simulink model "Pacemaker_Deliverable_1"  (R2025a)
settings: Solver=FixedStepAuto  StartTime=0.0  StopTime=10.0  FixedStep=1e-3  RelTol=1e-3  EnableMultiTasking=on
undefined symbols (not defined in the file): D0, D1, D10, D11, D12, D13, D2, D3, D4, D5, D6, D7, D8, D9, PTA0, PTA1, PTA2, PTB23, PTB9, PTC16, PTC17, PTC2, PTC3, PTC4, PTD0, PTD1, PTD2, PTD3
libraries: frdmk64flib x15
settings Model: ExtModeTrigDuration=5  Creator=harry  LastModifiedBy=justi
settings SolverCC: AlgebraicLoopSolver=TrustRegion
settings OptimizationCC: EnhancedBackFolding=on  PassReuseOutputArgsAs=Individual arguments  ZeroExternalMemoryAtStartup=off  ZeroInternalMemoryAtStartup=off  MaxStackSize=64  OptimizeBlockOrder=speed  DifferentSizesBufferReuse=on  OptimizationCustomize=off  EfficientTunableParamExpr=on
settings DebuggingCC: ParameterTunabilityLossMsg=error  UnconnectedInputMsg=warning  UnconnectedOutputMsg=warning  UnconnectedLineMsg=warning
settings HardwareCC: ProdBitPerPointer=32.0  ProdBitPerSizeT=32.0  ProdBitPerPtrDiffT=32.0  ProdLargestAtomicInteger=Long  ProdLargestAtomicFloat=Double  ProdWordSize=32.0  ProdHWDeviceType=ARM Compatible->ARM Cortex
settings ModelReferenceCC: EnableRefExpFcnMdlSchedulingChecks=on
settings SFSimCC: MATLABDynamicMemAlloc=off
settings RTWCC: SystemTargetFile=ert.tlc  HardwareBoard=NXP FRDM-K64F  TLCOptions="-aInlineSetEventsForThisBaseRateFcn=TLC_FALSE -aSuppressMultiTaskScheduler=TLC_FALSE  -aRateBasedStepFcn=0"  TemplateMakefile=ert_default_tmf  Toolchain=GNU Tools for ARM Embedded Processors  GPUComputeCapability=3.5  Description=Embedded Coder
settings CodeAppCC: ForceParamTrailComments=on  IgnoreCustomStorageClasses=off  OperatorAnnotations=on  SimulinkDataObjDesc=on  SFDataObjDesc=on  InsertBlockDesc=on
settings ERTTargetCC: ExtModeTransport=0.0  ExtModeStaticAlloc=off  ExtModeMexFile=ext_comm  ExtModeIntrfLevel=Level1  InlinedParameterPlacement=Hierarchical  DynamicArrayContainerType=coder::array

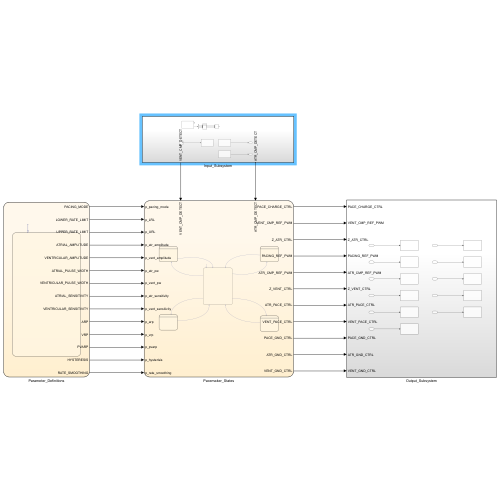
[thumbnail: Simulink's stored preview of the top-level diagram]
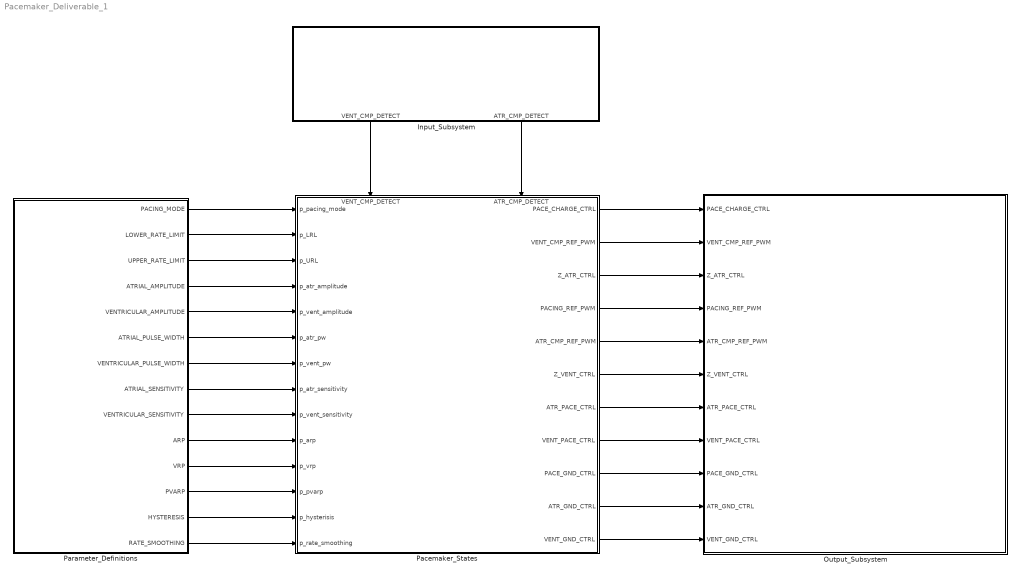
== system Pacemaker_Deliverable_1 ==
  Input_Subsystem : Subsystem
      settings: PortSchema="{\"entries\":[{\"content\":{\"sides\":[{\"content\":{\"connectorIds\":[]},\"type\":\"ConnectorPlacement.EquallySpacedRectSide\",\"uuid\":\"7aa35272-78af-4b86-b792-d4552822e5cd\"},{\"content\":{\"connectorIds\":[],\"side\":\"RIGHT\"},\"type\":\"ConnectorPlacement.EquallySpacedRectSide\",\"uuid\":\"1eeedbdd-e182-4d72-ab10-92c9b2e47973\"},{\"content\":{\"connectorIds\":[],\"side\":\"TOP\"},\"type\":\"ConnectorPlacement.EquallySpacedRectSide\",\"uuid\":\"983587ba-d25a-459a-9a3e-9f5267716506\"},{\"content\":{\"connectorIds\":[\"Out1\",\"Out2\"],\"side\":\"BOTTOM\"},\"type\":\"ConnectorPlacement.EquallySpacedRectSide\",\"uuid\":\"0cdd1530-a104-439a-8a9c-6ed3bc5e5b37\"}]},\"type\":\"ConnectorPlacement.EquallySpacedConnector\",\"uuid\":\"2c1020c0-9cac-4181-8f0f-8201f6fe3f1b\"}],\"packageUris\":[\"http://schema.mathworks.com/mf0/Connector/19700101\"],\"version\":\"1.0\"}"
  Output_Subsystem : Subsystem
  Pacemaker_States : Stateflow chart  TreatAsAtomicUnit=on
      settings: PortSchema="{\"entries\":[{\"content\":{\"sides\":[{\"content\":{\"connectorIds\":[\"In8\",\"In4\",\"In14\",\"In6\",\"In3\",\"In7\",\"In5\",\"In12\",\"In13\",\"In10\",\"In11\",\"In16\",\"In9\",\"In15\"]},\"type\":\"ConnectorPlacement.EquallySpacedRectSide\",\"uuid\":\"f7c19d4e-8469-492c-a227-d3ddaf8b11c5\"},{\"content\":{\"connectorIds\":[\"Out8\",\"Out10\",\"Out1\",\"Out7\",\"Out11\",\"Out2\",\"Out3\",\"Out4\",\"Out9\",\"Out5\",\"Out6\"],\"side\":\"RIGHT\"},\"type\":\"ConnectorPlacement.EquallySpacedRectSide\",\"uuid\":\"dec5cef5-f41f-4673-aab9-f0ca8e60eeee\"},{\"content\":{\"connectorIds\":[\"In1\",\"In2\"],\"side\":\"TOP\"},\"type\":\"ConnectorPlacement.EquallySpacedRectSide\",\"uuid\":\"d69c500f-a27d-47d0-a981-29ab2c08cb35\"}]},\"type\":\"ConnectorPlacement.EquallySpacedConnector\",\"uuid\":\"10b708de-b80e-4994-a949-6ddae67c2dfd\"}],\"packageUris\":[\"http://schema.mathworks.com/mf0/Connector/19700101\"],\"version\":\"1.0\"}"
  Parameter_Definitions : Stateflow chart  TreatAsAtomicUnit=on
      settings: PortSchema="{\"entries\":[{\"content\":{\"sides\":[{\"content\":{\"connectorIds\":[]},\"type\":\"ConnectorPlacement.EquallySpacedRectSide\",\"uuid\":\"6604c324-2550-41c6-b2f2-71f3c706ced3\"},{\"content\":{\"connectorIds\":[\"Out1\",\"Out2\",\"Out3\",\"Out4\",\"Out7\",\"Out5\",\"Out9\",\"Out8\",\"Out6\",\"Out14\",\"Out13\",\"Out12\",\"Out11\",\"Out10\"],\"side\":\"RIGHT\"},\"type\":\"ConnectorPlacement.EquallySpacedRectSide\",\"uuid\":\"7ef386a9-7013-4033-b302-df52cb7a11b5\"},{\"content\":{\"connectorIds\":[],\"side\":\"TOP\"},\"type\":\"ConnectorPlacement.EquallySpacedRectSide\",\"uuid\":\"6c75a8fc-d552-4f9b-9a9a-6aef7cb72f4d\"}]},\"type\":\"ConnectorPlacement.EquallySpacedConnector\",\"uuid\":\"c0dbf2bf-9097-47f1-93b4-de483c75bb4c\"}],\"packageUris\":[\"http://schema.mathworks.com/mf0/Connector/19700101\"],\"version\":\"1.0\"}"
  wires:
  Pacemaker_States/8(PACE_CHARGE_CTRL) -> Output_Subsystem/1(PACE_CHARGE_CTRL)
  Pacemaker_States/10(VENT_CMP_REF_PWM) -> Output_Subsystem/2(VENT_CMP_REF_PWM)
  Pacemaker_States/1(Z_ATR_CTRL) -> Output_Subsystem/3(Z_ATR_CTRL)
  Pacemaker_States/7(PACING_REF_PWM) -> Output_Subsystem/4(PACING_REF_PWM)
  Pacemaker_States/11(ATR_CMP_REF_PWM) -> Output_Subsystem/5(ATR_CMP_REF_PWM)
  Pacemaker_States/2(Z_VENT_CTRL) -> Output_Subsystem/6(Z_VENT_CTRL)
  Pacemaker_States/3(ATR_PACE_CTRL) -> Output_Subsystem/7(ATR_PACE_CTRL)
  Pacemaker_States/4(VENT_PACE_CTRL) -> Output_Subsystem/8(VENT_PACE_CTRL)
  Pacemaker_States/9(PACE_GND_CTRL) -> Output_Subsystem/9(PACE_GND_CTRL)
  Pacemaker_States/5(ATR_GND_CTRL) -> Output_Subsystem/10(ATR_GND_CTRL)
  Pacemaker_States/6(VENT_GND_CTRL) -> Output_Subsystem/11(VENT_GND_CTRL)
  Input_Subsystem/1(VENT_CMP_DETECT) -> Pacemaker_States/1(VENT_CMP_DETECT)
  Input_Subsystem/2(ATR_CMP_DETECT) -> Pacemaker_States/2(ATR_CMP_DETECT)
  Parameter_Definitions/1(PACING_MODE) -> Pacemaker_States/8(p_pacing_mode)
  Parameter_Definitions/2(LOWER_RATE_LIMIT) -> Pacemaker_States/4(p_LRL)
  Parameter_Definitions/4(ATRIAL_AMPLITUDE) -> Pacemaker_States/6(p_atr_amplitude)
  Parameter_Definitions/7(VENTRICULAR_AMPLITUDE) -> Pacemaker_States/3(p_vent_amplitude)
  Parameter_Definitions/5(ATRIAL_PULSE_WIDTH) -> Pacemaker_States/7(p_atr_pw)
  Parameter_Definitions/9(VENTRICULAR_PULSE_WIDTH) -> Pacemaker_States/5(p_vent_pw)
  Parameter_Definitions/14(ARP) -> Pacemaker_States/10(p_arp)
  Parameter_Definitions/13(VRP) -> Pacemaker_States/11(p_vrp)
  Parameter_Definitions/11(HYSTERESIS) -> Pacemaker_States/9(p_hysterisis)
  Parameter_Definitions/10(RATE_SMOOTHING) -> Pacemaker_States/15(p_rate_smoothing)
  Parameter_Definitions/8(ATRIAL_SENSITIVITY) -> Pacemaker_States/12(p_atr_sensitivity)
  Parameter_Definitions/6(VENTRICULAR_SENSITIVITY) -> Pacemaker_States/13(p_vent_sensitivity)
  Parameter_Definitions/3(UPPER_RATE_LIMIT) -> Pacemaker_States/14(p_URL)
  Parameter_Definitions/12(PVARP) -> Pacemaker_States/16(p_pvarp)

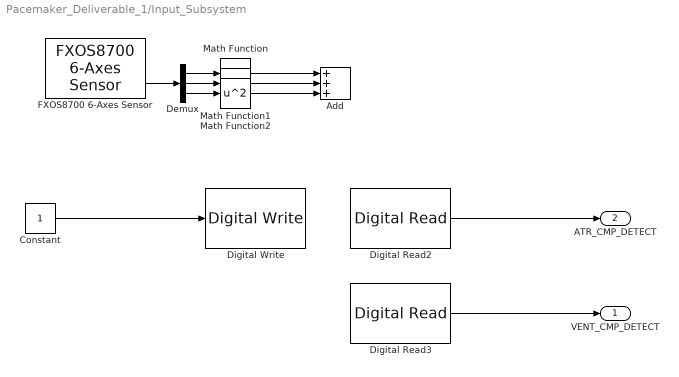
== system Pacemaker_Deliverable_1/Input_Subsystem ==
  Add : Sum  Inputs=+++
  Constant : Constant
  Demux : Demux  Outputs=3
  Digital Read2 : frdmk64flib/Digital Read  Whichpin=PTC16 (D0)  SampleTime=-1
  Digital Read3 : frdmk64flib/Digital Read  Whichpin=PTC17 (D1)  SampleTime=-1
  Digital Write : frdmk64flib/Digital Write  Whichpin=PTD1 (D13)
  FXOS8700 6-Axes Sensor : frdmk64flib/FXOS8700 6-Axes Sensor  Activesensor=Accelerometer and Magnetometer  ODR=800Hz  HybridODR=400Hz  Accelfullrange=-4g to +4g  SampleTime=-1
  Math Function : Math  Operator=square
  Math Function1 : Math  Operator=square
  Math Function2 : Math  Operator=square
  VENT_CMP_DETECT : Outport
  ATR_CMP_DETECT : Outport  Port=2
  wires:
  Constant/1 -> Digital Write/1
  Digital Read2/1 -> ATR_CMP_DETECT/1
  Digital Read3/1 -> VENT_CMP_DETECT/1
  FXOS8700 6-Axes Sensor/2 -> Demux/1
  Demux/1 -> Math Function/1
  Demux/2 -> Math Function1/1
  Demux/3 -> Math Function2/1
  Math Function/1 -> Add/1
  Math Function1/1 -> Add/2
  Math Function2/1 -> Add/3

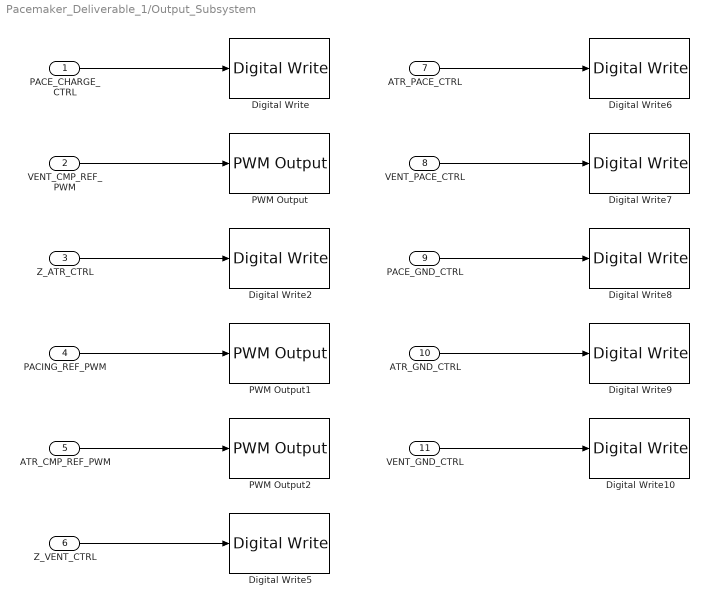
== system Pacemaker_Deliverable_1/Output_Subsystem ==
  PACE_CHARGE_CTRL : Inport
  VENT_CMP_REF_PWM : Inport  Port=2
  Z_ATR_CTRL : Inport  Port=3
  PACING_REF_PWM : Inport  Port=4
  ATR_CMP_REF_PWM : Inport  Port=5
  Z_VENT_CTRL : Inport  Port=6
  ATR_PACE_CTRL : Inport  Port=7
  VENT_PACE_CTRL : Inport  Port=8
  PACE_GND_CTRL : Inport  Port=9
  ATR_GND_CTRL : Inport  Port=10
  VENT_GND_CTRL : Inport  Port=11
  Digital Write : frdmk64flib/Digital Write  Whichpin=PTB9 (D2)
  Digital Write10 : frdmk64flib/Digital Write  Whichpin=PTD3 (D12)
  Digital Write2 : frdmk64flib/Digital Write  Whichpin=PTB23 (D4)
  Digital Write5 : frdmk64flib/Digital Write  Whichpin=PTC3 (D7)
  Digital Write6 : frdmk64flib/Digital Write  Whichpin=PTA0 (D8)
  Digital Write7 : frdmk64flib/Digital Write  Whichpin=PTC4 (D9)
  Digital Write8 : frdmk64flib/Digital Write  Whichpin=PTD0 (D10)
  Digital Write9 : frdmk64flib/Digital Write  Whichpin=PTD2 (D11)
  PWM Output : frdmk64flib/PWM Output  Whichpin=PTA1 (D3)  InitialFrequency=2000  InitialDutyCycle=0
  PWM Output1 : frdmk64flib/PWM Output  Whichpin=PTA2 (D5)  InitialFrequency=2000  InitialDutyCycle=0
  PWM Output2 : frdmk64flib/PWM Output  Whichpin=PTC2 (D6)  InitialFrequency=2000  InitialDutyCycle=0
  wires:
  PACE_CHARGE_CTRL/1 -> Digital Write/1
  VENT_CMP_REF_PWM/1 -> PWM Output/1
  Z_ATR_CTRL/1 -> Digital Write2/1
  ATR_CMP_REF_PWM/1 -> PWM Output2/1
  Z_VENT_CTRL/1 -> Digital Write5/1
  PACING_REF_PWM/1 -> PWM Output1/1
  VENT_PACE_CTRL/1 -> Digital Write7/1
  ATR_GND_CTRL/1 -> Digital Write9/1
  PACE_GND_CTRL/1 -> Digital Write8/1
  ATR_PACE_CTRL/1 -> Digital Write6/1
  VENT_GND_CTRL/1 -> Digital Write10/1

== stateflow chart Pacemaker_Deliverable_1/Pacemaker_States ==
  state VOO
    entry:
    state Discharge_VOO
      entry:
      %pacing state 3
      PACE_GND_CTRL=1;
      VENT_PACE_CTRL=0;
      VENT_GND_CTRL=1;
      %pacing state 1
      PACING_REF_PWM= VOO_amp;
      PACE_CHARGE_CTRL=1;
    state Initial_VOO
      entry:
      %This is the initial state to define
      %varriables that wont change
      discharge_time = ((60/p_LRL)*1000)-p_vent_pw;
      VOO_amp = (p_vent_amplitude/5000)*100;
      ATR_PACE_CTRL=0;
      ATR_GND_CTRL= 0;
      Z_ATR_CTRL=0;
      Z_VENT_CTRL=0;
    state Charge_VOO
      entry:
      %pacing state 2
      PACE_CHARGE_CTRL=0;
      PACE_GND_CTRL=1;
      VENT_GND_CTRL=0;
      VENT_PACE_CTRL=1;
    (default) -> Initial_VOO
    Initial_VOO -> Discharge_VOO
    Discharge_VOO -> Charge_VOO : [after(discharge_time, msec)]
    Charge_VOO -> Discharge_VOO : [after(p_vent_pw, msec)]
  state AOO
    entry:
    state Discharge_AOO
      entry:
      %pacing state 3
      PACE_GND_CTRL=1;
      ATR_PACE_CTRL=0;
      ATR_GND_CTRL=1;
      %pacing state 1
      PACING_REF_PWM= AOO_amp;
      PACE_CHARGE_CTRL=1;
    state Initial_AOO
      entry:
      %Defining variables
      discharge_time = ((60/p_LRL)*1000)-p_atr_pw;
      AOO_amp = (p_atr_amplitude/5000)*100;
      Z_VENT_CTRL=0;
      VENT_GND_CTRL=0;
      VENT_PACE_CTRL=0;
      Z_ATR_CTRL=0;
    state Charge_AOO
      entry:
      %pacing state 2
      PACE_CHARGE_CTRL=0;
      PACE_GND_CTRL=1;
      ATR_GND_CTRL= 0;
      ATR_PACE_CTRL=1;
    (default) -> Initial_AOO
    Initial_AOO -> Discharge_AOO
    Discharge_AOO -> Charge_AOO : [after(discharge_time, msec)]
    Charge_AOO -> Discharge_AOO : [after(p_atr_pw, msec)]
  state Initial_State
    entry:
    VENT_CMP_REF_PWM = 52;
    ATR_CMP_REF_PWM = 51;
  state VVI
    entry:
    state Discharge_VVI
      entry:
      %pacing state 3
      PACE_GND_CTRL=1;
      VENT_PACE_CTRL=0;
      VENT_GND_CTRL=1;
      % pacing state 1
      PACING_REF_PWM= VVI_amp;
      PACE_CHARGE_CTRL=1;
    state Initial_VVI
      entry:
      %Initial state defining variables
      discharge_time = ((60/p_LRL)*1000)-p_vent_pw;
      VVI_amp = (p_vent_amplitude/5000)*100;
      ATR_PACE_CTRL=0;
      ATR_GND_CTRL= 0;
      Z_ATR_CTRL=0;
      Z_VENT_CTRL=0;
    state Charge_VVI
      entry:
      %pacing state 2
      PACE_CHARGE_CTRL=0;
      PACE_GND_CTRL=1;
      VENT_GND_CTRL=0;
      VENT_PACE_CTRL=1;
    (default) -> Initial_VVI
    Initial_VVI -> Discharge_VVI
    Discharge_VVI -> (junction 38)
    (junction 38) -> Discharge_VVI [order 2] : [VENT_CMP_DETECT == true]
    Charge_VVI -> Discharge_VVI : [after(p_vent_pw, msec)]
    (junction 38) -> Charge_VVI [order 1] : [after(discharge_time, msec) && VENT_CMP_DETECT == false]
  state AAI
    entry:
    state Discharge_AAI
      entry:
      %pacing state 3
      PACE_GND_CTRL=1;
      ATR_PACE_CTRL=0;
      ATR_GND_CTRL=1;
      %pacing state 1
      PACING_REF_PWM= AAI_amp;
      PACE_CHARGE_CTRL=1;
    state Initial_AAI
      entry:
      %initial state defining variables
      discharge_time = ((60/p_LRL)*1000)-p_atr_pw;
      AAI_amp = (p_atr_amplitude/5000)*100;
      Z_VENT_CTRL=0;
      VENT_GND_CTRL=0;
      VENT_PACE_CTRL=0;
      Z_ATR_CTRL=0;
    state Charge_AAI
      entry:
      %pacing state 2
      PACE_CHARGE_CTRL=0;
      PACE_GND_CTRL=1;
      ATR_GND_CTRL= 0;
      ATR_PACE_CTRL=1;
    (default) -> Initial_AAI
    Initial_AAI -> Discharge_AAI
    Discharge_AAI -> (junction 45)
    (junction 45) -> Discharge_AAI [order 2] : [ATR_CMP_DETECT == true]
    Charge_AAI -> Discharge_AAI : [after(p_atr_pw, msec)]
    (junction 45) -> Charge_AAI [order 1] : [after(discharge_time , msec) && ATR_CMP_DETECT == false]
  AOO -> Initial_State : [p_pacing_mode ~= 2]
  VOO -> Initial_State : [p_pacing_mode ~= 1]
  Initial_State -> VOO [order 1] : [p_pacing_mode == 1]
  Initial_State -> AOO [order 2] : [p_pacing_mode == 2]
  (default) -> Initial_State
  Initial_State -> VVI [order 4] : [p_pacing_mode == 4]
  Initial_State -> AAI [order 3] : [p_pacing_mode == 3]
  VVI -> Initial_State : [p_pacing_mode ~=  4]
  AAI -> Initial_State : [p_pacing_mode ~= 3]
  data: Z_ATR_CTRL output; Z_VENT_CTRL output; ATR_PACE_CTRL output; VENT_PACE_CTRL output; ATR_GND_CTRL output; VENT_GND_CTRL output; PACING_REF_PWM output; PACE_CHARGE_CTRL output; PACE_GND_CTRL output; VENT_CMP_REF_PWM output; ATR_CMP_REF_PWM output; VENT_CMP_DETECT input; ATR_CMP_DETECT input; p_vent_amplitude input; p_LRL input; p_vent_pw input; p_atr_amplitude input; p_atr_pw input; p_pacing_mode input; p_hysterisis input; p_arp input; p_vrp input; p_atr_sensitivity input; p_vent_sensitivity input; p_URL input; p_rate_smoothing input; p_pvarp input; discharge_time local; VOO_amp local; AOO_amp local; VVI_amp local; AAI_amp local

== stateflow chart Pacemaker_Deliverable_1/Parameter_Definitions ==
  state Parameter_Definitions
    entry:
    %Defining the initial paramater values
    PACING_MODE = 1;
    LOWER_RATE_LIMIT = 60;
    UPPER_RATE_LIMIT = 120;
    ATRIAL_AMPLITUDE = 3500;
    VENTRICULAR_AMPLITUDE = 3500;
    ATRIAL_PULSE_WIDTH = 0.4;
    VENTRICULAR_PULSE_WIDTH = 0.4;
    ATRIAL_SENSITIVITY = 2.75;
    VENTRICULAR_SENSITIVITY = 2.5;
    ARP = 250;
    VRP = 320;
    PVARP = 250;
    HYSTERESIS = false;
    RATE_SMOOTHING = false;
    MAX_SENSOR_RATE = 120;
    ACTIVITY_THRESHOLD = 4;
    RESPONSE_FACTOR = 8;
    REACTION_TIME = 25;
    RECOVERY_TIME = 8;
  (default) -> Parameter_Definitions
  data: PACING_MODE output; LOWER_RATE_LIMIT output; UPPER_RATE_LIMIT output; ATRIAL_AMPLITUDE output; ATRIAL_PULSE_WIDTH output; VENTRICULAR_SENSITIVITY output; VENTRICULAR_AMPLITUDE output; ATRIAL_SENSITIVITY output; VENTRICULAR_PULSE_WIDTH output; RATE_SMOOTHING output; HYSTERESIS output; PVARP output; VRP output; ARP output
